simulink model "Kinematics"  (R2024a)
settings: Solver=VariableStepAuto  StartTime=0.0  StopTime=10.0  RelTol=1e-3
undefined symbols (not defined in the file or in its folder): fractalcoef, robotGoal, startPose
libraries: mspsensorlib x1, mspfiltlib x1, robotmobilelib x1
settings Model: DataDictionary=VIPR_Arch_v2_dict.sldd  Creator=charber  LastModifiedBy=jkcolem
settings ModelReferenceCC: ModelReferenceMinAlgLoopOccurrences=on

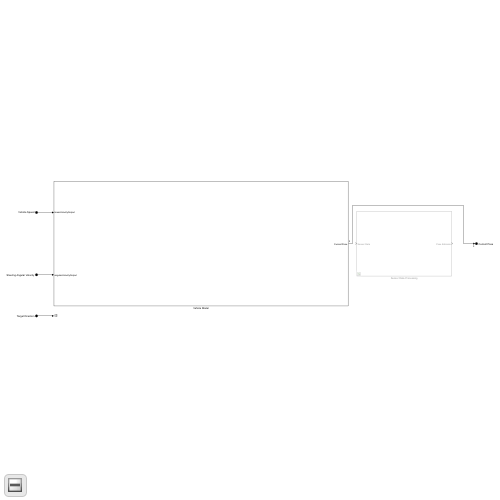
[thumbnail: Simulink's stored preview of the top-level diagram]
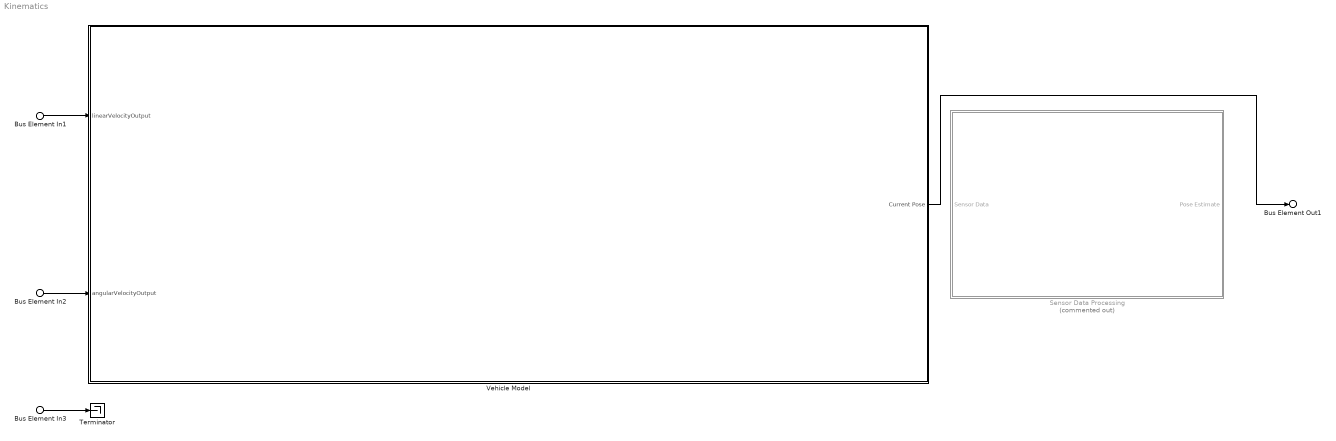
== system Kinematics ==
  Bus Element In1 : Inport  PortName=Vehicle Speed
  Bus Element In2 : Inport  Port=2  PortName=Steering Angular Velocity
  Bus Element In3 : Inport  Port=3  PortName=Target Direction
  Sensor Data Processing : Subsystem  Commented=on
  Terminator : Terminator
  Vehicle Model : Subsystem
  Bus Element Out1 : Outport  PortName=Current Pose
  wires:
  Bus Element In3/1 -> Terminator/1
  Bus Element In1/1 -> Vehicle Model/1(linearVelocityOutput)
  Bus Element In2/1 -> Vehicle Model/2(angularVelocityOutput)
  Vehicle Model/1(Current Pose) -> Bus Element Out1/1

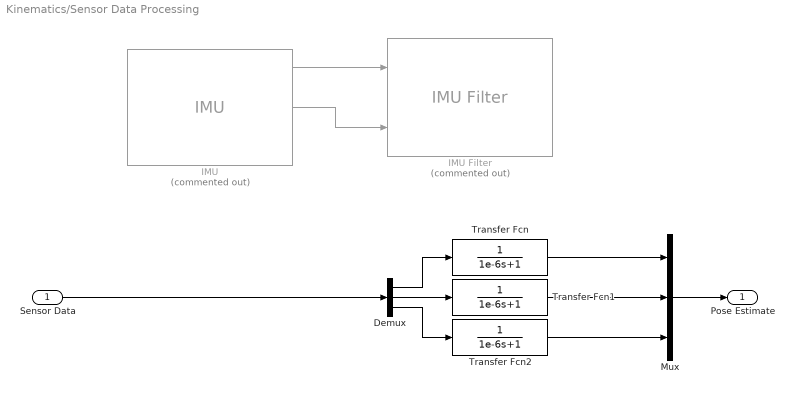
== system Kinematics/Sensor Data Processing ==
  Sensor Data : Inport
  Demux : Demux  Outputs=3
  IMU : mspsensorlib/IMU  Commented=on  DispRefFrame=NED  TemperaturePort=off  Temperature=25  MagneticFieldPort=off  MagneticFieldNED=[ 27.5550, -2.4169, -16.0849 ]  MagneticFieldENU=[ -2.4169, 27.5550, 16.0849 ]  SeedDouble=67  SimulateUsing=Interpreted execution  AccelParamsMeasurementRange=Inf  AccelParamsResolution=0  AccelParamsConstantBias=[ 0, 0, 0 ]  AccelParamsAxesMisalignment=[ 100, 0, 0; 0, 100, 0; 0, 0, 100 ]  AccelParamsNoiseDensity=[ 0, 0, 0 ]  AccelParamsBiasInstability=[ 0, 0, 0 ]  AccelParamsBiasInstabilityNumerator=fractalcoef().Numerator  AccelParamsBiasInstabilityDenominator=fractalcoef().Denominator  AccelParamsRandomWalk=[ 0, 0, 0 ]  AccelParamsNoiseType=double-sided  AccelParamsTemperatureBias=[ 0, 0, 0 ]  AccelParamsTemperatureScaleFactor=[ 0, 0, 0 ]  GyroParamsMeasurementRange=Inf  GyroParamsResolution=0  GyroParamsConstantBias=[ 0, 0, 0 ]  GyroParamsAxesMisalignment=[ 100, 0, 0; 0, 100, 0; 0, 0, 100 ]  GyroParamsAccelerationBias=[ 0, 0, 0 ]  GyroParamsNoiseDensity=[ 0, 0, 0 ]  GyroParamsBiasInstability=[ 0, 0, 0 ]  GyroParamsBiasInstabilityNumerator=fractalcoef().Numerator  GyroParamsBiasInstabilityDenominator=fractalcoef().Denominator  GyroParamsRandomWalk=[ 0, 0, 0 ]  GyroParamsNoiseType=double-sided  GyroParamsTemperatureBias=[ 0, 0, 0 ]  GyroParamsTemperatureScaleFactor=[ 0, 0, 0 ]  MagParamsMeasurementRange=Inf  MagParamsResolution=0  MagParamsConstantBias=[ 0, 0, 0 ]  MagParamsAxesMisalignment=[ 100, 0, 0; 0, 100, 0; 0, 0, 100 ]  MagParamsNoiseDensity=[ 0, 0, 0 ]  MagParamsBiasInstability=[ 0, 0, 0 ]  MagParamsBiasInstabilityNumerator=fractalcoef().Numerator  MagParamsBiasInstabilityDenominator=fractalcoef().Denominator  MagParamsRandomWalk=[ 0, 0, 0 ]  MagParamsNoiseType=double-sided  MagParamsTemperatureBias=[ 0, 0, 0 ]  MagParamsTemperatureScaleFactor=[ 0, 0, 0 ]
  IMU Filter : mspfiltlib/IMU Filter  Commented=on  DispRefFrame=NED  OrientationFormat=quaternion  DecimationFactor=1  InitialProcessNoise=imufilter.defaultProcessNoise  AccelerometerNoise=0.0001924722  GyroscopeNoise=9.1385e-5  GyroscopeDriftNoise=3.0462e-13  LinearAccelerationNoise=0.0096236100000000012  LinearAccelerationDecayFactor=0.5  SimulateUsing=Interpreted execution
  Mux : Mux  Inputs=3
  Transfer Fcn : TransferFcn  Denominator=[1e-6 1]
  Transfer Fcn1 : TransferFcn  Denominator=[1e-6 1]
  Transfer Fcn2 : TransferFcn  Denominator=[1e-6 1]
  Pose Estimate : Outport
  wires:
  IMU/2 -> IMU Filter/2
  IMU/1 -> IMU Filter/1
  Transfer Fcn/1 -> Mux/1
  Sensor Data/1 -> Demux/1
  Demux/1 -> Transfer Fcn/1
  Demux/2 -> Transfer Fcn1/1
  Transfer Fcn1/1 -> Mux/2
  Demux/3 -> Transfer Fcn2/1
  Transfer Fcn2/1 -> Mux/3
  Mux/1 -> Pose Estimate/1

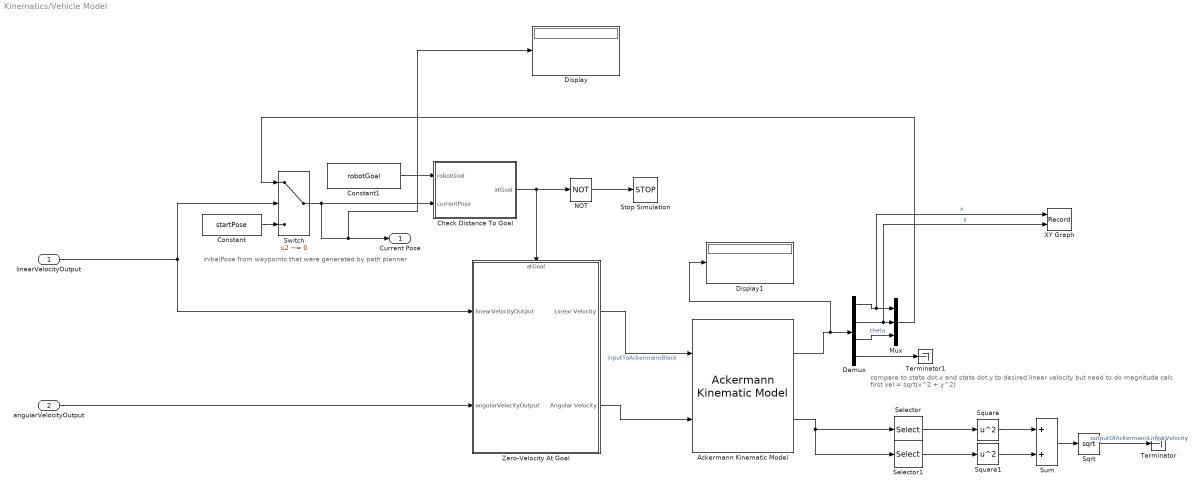
== system Kinematics/Vehicle Model ==
  note: initialPose from waypoints that were generated by path planner
  note: compare to state dot.x and state dot.y to desired linear velocity but need to do magnitude calc first vel = sqrt(x^2 + y^2)
  linearVelocityOutput : Inport
  angularVelocityOutput : Inport  Port=2
  Ackermann Kinematic Model : robotmobilelib/Ackermann Kinematic Model  WheelBase=1  VehicleSpeedRange=[-inf inf]  MaxSteeringAngle=pi/4  InitialState=[0; 0; 0; 0]  SimulateUsing=Interpreted execution
  Check Distance To Goal : Subsystem
  Constant : Constant  Value=startPose
  Constant1 : Constant  Value=robotGoal
  Demux : Demux
  Display : Display
  Display1 : Display
  Mux : Mux  Inputs=3
  NOT : Logic  Operator=NOT  IconShape=distinctive  AllPortsSameDT=off  OutDataTypeStr=boolean
  Selector : Selector  InputPortWidth=4  IndexOptions=Index vector (dialog)  Indices=[1]  OutputSizes=1
  Selector1 : Selector  InputPortWidth=4  IndexOptions=Index vector (dialog)  Indices=[2]  OutputSizes=1
  Sqrt : Sqrt
  Square : Math  Operator=square
  Square1 : Math  Operator=square
  Stop Simulation : Stop
  Sum : Sum
  Switch : Switch  Criteria=u2 ~= 0  SaturateOnIntegerOverflow=off  InputSameDT=off
  Terminator : Terminator
  Terminator1 : Terminator
  XY Graph : Record  FileSettingsInternal="{\"entries\":[{\"content\":{\"excelSettings\":{\"content\":{},\"type\":\"Streamout.ExcelSettings\"}},\"type\":\"Streamout.FileSettingStorage\",\"uuid\":\"\"}],\"packageUris\":[\"http:\\/\\/schema.mathworks.com\\/mf0\\/streamout_blocks\\/R2020a\"],\"version\":\"1.0\"}"  Layout=[1 1]  SignalsInternal="{\"entries\":[{\"content\":{\"signals\":[{\"content\":{\"blockPath\":[],\"dimensions\":[1],\"domain\":\"\",\"lineColor\":\"#139fff\",\"lineWidth\":2,\"port\":1,\"sid\":[\"\",\"\"],\"signalID\":1,\"signalName\":\"x\"},\"type\":\"RecordBlkView.Signal\",\"uuid\":\"\"},{\"content\":{\"blockPath\":[],\"dimensions\":[1],\"domain\":\"\",\"lineColor\":\"#ff6929\",\"lineWidth\":2,\"port\":2,\"sid\":[\"\",\"\"],\"signalID\":2,\"signalName\":\"y\"},\"type\":\"RecordBlkView.Signal\",\"uuid\":\"\"}]},\"type\":\"RecordBlkView.InputSignals\",\"uuid\":\"\"},{\"content\":{\"signals\":[{\"content\":{\"blockPath\":[],\"dimensions\":[1],\"domain\":\"\",\"lineColor\":\"#139fff\",\"lineWidth\":2,\"port\":1,\"sid\":[\"\",\"\"],\"signalID\":1,\"signalName\":\"x\"},\"type\":\"RecordBlkView.Signal\",\"uuid\":\"\"},{\"content\":{\"blockPath\":[],\"dimensions\":[1],\"domain\":\"\",\"lineColor\":\"#ff6929\",\"lineWidth\":2,\"plots\":[ 1 ],\"port\":2,\"sid\":[\"\",\"\"],\"signalID\":2,\"signalName\":\"y\"},\"type\":\"RecordBlkView.Signal\",\"uuid\":\"\"}]},\"type\":\"RecordBlkView.InputSignals\",\"uuid\":\"\"}],\"packageUris\":[\"http:\\/\\/schema.mathworks.com\\/mf0\\/streamout_blocks\\/R2020a\"],\"version\":\"1.0\"}"  VisualizationBindings="{\"xyplotplugin\":{\"info\":[{\"series\":[{\"bindingParametersList\":[{\"parameter\":\"X-Axis\",\"signalID\":4152,\"signalName\":\"XY Graph:1\"},{\"parameter\":\"Y-Axis\",\"signalID\":4155,\"signalName\":\"XY Graph:2\"}],\"seriesID\":0}],\"subplotID\":1}]}}"  CompatibilityTag=XY
  Zero-Velocity At Goal : Subsystem
      settings: PortSchema="{\"entries\":[{\"content\":{\"sides\":[{\"content\":{\"connectorIds\":[\"In1\",\"In2\"]},\"type\":\"ConnectorPlacement.EquallySpacedRectSide\",\"uuid\":\"d6ef090c-8691-4f8e-808e-16a05b1c931f\"},{\"content\":{\"connectorIds\":[\"Out1\",\"Out2\"],\"side\":\"RIGHT\"},\"type\":\"ConnectorPlacement.EquallySpacedRectSide\",\"uuid\":\"2ae6408e-e944-4e5d-bf23-2707e82d0ba7\"},{\"content\":{\"connectorIds\":[\"In3\"],\"side\":\"TOP\"},\"type\":\"ConnectorPlacement.EquallySpacedRectSide\",\"uuid\":\"29270005-91b8-4dcb-ad7c-17893aa9f4c0\"}]},\"type\":\"ConnectorPlacement.EquallySpacedConnector\",\"uuid\":\"a9fc078d-7ce2-488f-9666-d3d979ba1bbe\"}],\"packageUris\":[\"http://schema.mathworks.com/mf0/Connector/R2020b\"],\"version\":\"1.0\"}"
  Current Pose : Outport
  wires:
  angularVelocityOutput/1 -> Zero-Velocity At Goal/2(angularVelocityOutput)
  Demux/4 -> Terminator1/1
  Demux/2 -> XY Graph/2, Mux/2  "y"
  Mux/1 -> Switch/1
  Demux/3 -> Mux/3  "theta"
  linearVelocityOutput/1 -> Switch/2, Zero-Velocity At Goal/1(linearVelocityOutput)
  Switch/1 -> Display/1, Current Pose/1, Check Distance To Goal/2(currentPose)
  Check Distance To Goal/1(atGoal) -> Zero-Velocity At Goal/3(atGoal), NOT/1
  Constant/1 -> Switch/3
  Ackermann Kinematic Model/1 -> Display1/1, Demux/1
  Constant1/1 -> Check Distance To Goal/1(robotGoal)
  Zero-Velocity At Goal/1(Linear Velocity) -> Ackermann Kinematic Model/1  "inputToAckermannBlock"
  Demux/1 -> XY Graph/1, Mux/1  "x"
  NOT/1 -> Stop Simulation/1
  Zero-Velocity At Goal/2(Angular Velocity) -> Ackermann Kinematic Model/2
  Ackermann Kinematic Model/2 -> Selector1/1, Selector/1
  Selector/1 -> Square/1
  Selector1/1 -> Square1/1
  Square/1 -> Sum/1
  Square1/1 -> Sum/2
  Sum/1 -> Sqrt/1
  Sqrt/1 -> Terminator/1  "outputOfAckermannLinearVelocity"

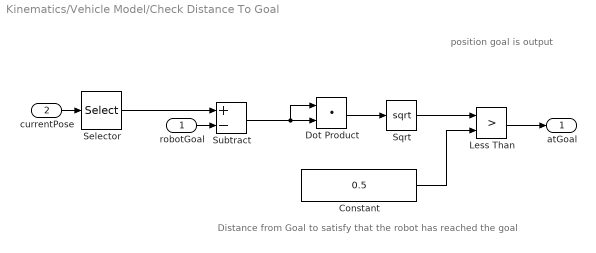
== system Kinematics/Vehicle Model/Check Distance To Goal ==
  note: Distance from Goal to satisfy that the robot has reached the goal
  note: position goal is output
  robotGoal : Inport
  currentPose : Inport  Port=2
  Constant : Constant  Value=0.5
  Dot Product : DotProduct  OutDataTypeStr=Inherit: Inherit via internal rule
  Less Than : RelationalOperator  Operator=>  OutDataTypeStr=boolean  RndMeth=Simplest  InputSameDT=off
  Selector : Selector  InputPortWidth=3  IndexOptions=Index vector (dialog)  Indices=[1 2]  OutputSizes=1
  Sqrt : Sqrt
  Subtract : Sum  Inputs=+-
  atGoal : Outport
  wires:
  robotGoal/1 -> Subtract/2
  Dot Product/1 -> Sqrt/1
  Constant/1 -> Less Than/2
  currentPose/1 -> Selector/1
  Less Than/1 -> atGoal/1
  Sqrt/1 -> Less Than/1
  Subtract/1 -> Dot Product/1, Dot Product/2
  Selector/1 -> Subtract/1

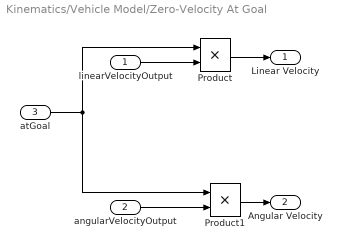
== system Kinematics/Vehicle Model/Zero-Velocity At Goal ==
  linearVelocityOutput : Inport
  angularVelocityOutput : Inport  Port=2
  atGoal : Inport  Port=3
  Product : Product
  Product1 : Product
  Linear Velocity : Outport  OutDataTypeStr=double
  Angular Velocity : Outport  Port=2  OutDataTypeStr=double
  wires:
  atGoal/1 -> Product1/1, Product/1
  angularVelocityOutput/1 -> Product1/2
  linearVelocityOutput/1 -> Product/2
  Product/1 -> Linear Velocity/1
  Product1/1 -> Angular Velocity/1
